simulink model "gm_PWMdutyFreqDetection"  (R2020b)
settings: Solver=FixedStepDiscrete  StartTime=0.0  StopTime=300e-6  RelTol=1e-3
libraries: simulink x4, hdlsllib x1
settings Model: Creator=Michael Hoerner  LastModifiedBy=Michael Hoerner
settings DataIOCC: LimitDataPoints=on  SaveOutput=off  SaveTime=off  ReturnWorkspaceOutputs=off
settings OptimizationCC: BlockReduction=off  ConditionallyExecuteInputs=off  DefaultParameterBehavior=Inlined  LifeSpan=inf
settings DebuggingCC: AlgebraicLoopMsg=error  InheritedTsInSrcMsg=none  SingleTaskRateTransMsg=warning  AllowSymbolicDim=off  StrictBusMsg=ErrorOnBusTreatedAsVector  SFUnexpectedBacktrackingDiag=warning  SFNoUnconditionalDefaultTransitionDiag=warning  SFExecutionAtInitializationDiag=none  ArithmeticOperatorsInVariantConditions=warning
settings HardwareCC: ProdBitPerPointer=32  ProdBitPerSizeT=32  ProdBitPerPtrDiffT=32  ProdLargestAtomicFloat=None  ProdIntDivRoundTo=Undefined  ProdEndianess=Unspecified  ProdWordSize=32  ProdHWDeviceType=ASIC/FPGA->ASIC/FPGA  ProdEqTarget=off
settings SFSimCC: SimUseLocalCustomCode=off  CustomCodeUndefinedFunction=UseInterfaceOnly
settings RTWCC: RTWUseLocalCustomCode=off
settings CodeAppCC: StateflowObjectComments=on
settings GRTTargetCC: TargetLangStandard=C89/C90 (ANSI)
settings ConfigComp: CovScope=ReferencedModels  CovMetricSettings=dw  CovSaveCumulativeToWorkspaceVar=on  CovSaveSingleToWorkspaceVar=on  CovExternalEMLEnable=off  CovSFcnEnable=off

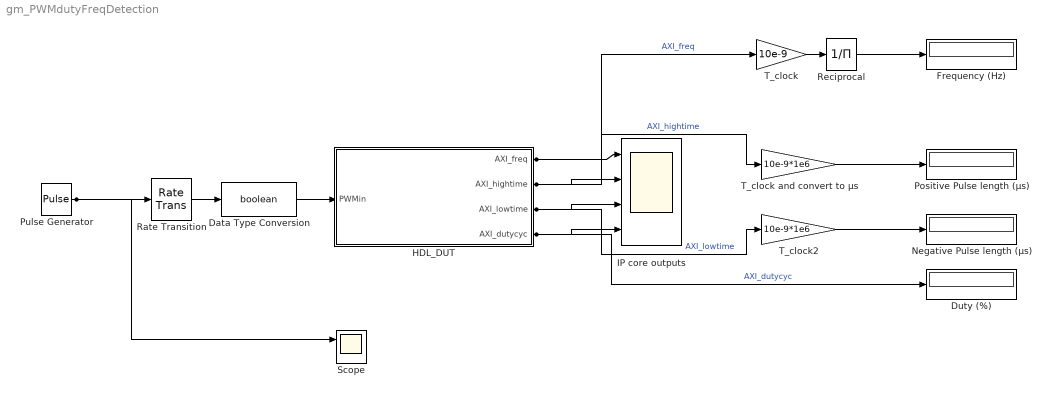
== system gm_PWMdutyFreqDetection ==
  Data Type Conversion : DataTypeConversion  OutDataTypeStr=boolean
  Duty (%) : Display
  Frequency (Hz) : Display
  HDL_DUT : Subsystem  TreatAsAtomicUnit=on
  IP core outputs : Scope  NumInputPorts=4
  Negative Pulse length (µs) : Display
  Positive Pulse length (µs) : Display
  Pulse Generator : DiscretePulseGenerator  PulseType=Time based  Period=1/10000  PulseWidth=25
  Rate Transition : RateTransition  OutPortSampleTime=10e-9
  Reciprocal : Product  Inputs=/
  Scope : Scope  NumInputPorts=2
  T_clock : Gain  Gain=10e-9
  T_clock and convert to µs : Gain  Gain=10e-9*1e6
  T_clock2 : Gain  Gain=10e-9*1e6
  wires:
  T_clock2/1 -> Negative Pulse length (µs)/1
  T_clock and convert to µs/1 -> Positive Pulse length (µs)/1
  Reciprocal/1 -> Frequency (Hz)/1
  T_clock/1 -> Reciprocal/1
  Data Type Conversion/1 -> HDL_DUT/1(PWMin)
  HDL_DUT/4(AXI_dutycyc) -> Duty (%)/1, IP core outputs/4  "AXI_dutycyc"
  HDL_DUT/3(AXI_lowtime) -> T_clock2/1, IP core outputs/3  "AXI_lowtime"
  HDL_DUT/2(AXI_hightime) -> IP core outputs/2, T_clock and convert to µs/1  "AXI_hightime"
  HDL_DUT/1(AXI_freq) -> IP core outputs/1, T_clock/1  "AXI_freq"
  Pulse Generator/1 -> Rate Transition/1, Scope/1
  Rate Transition/1 -> Data Type Conversion/1

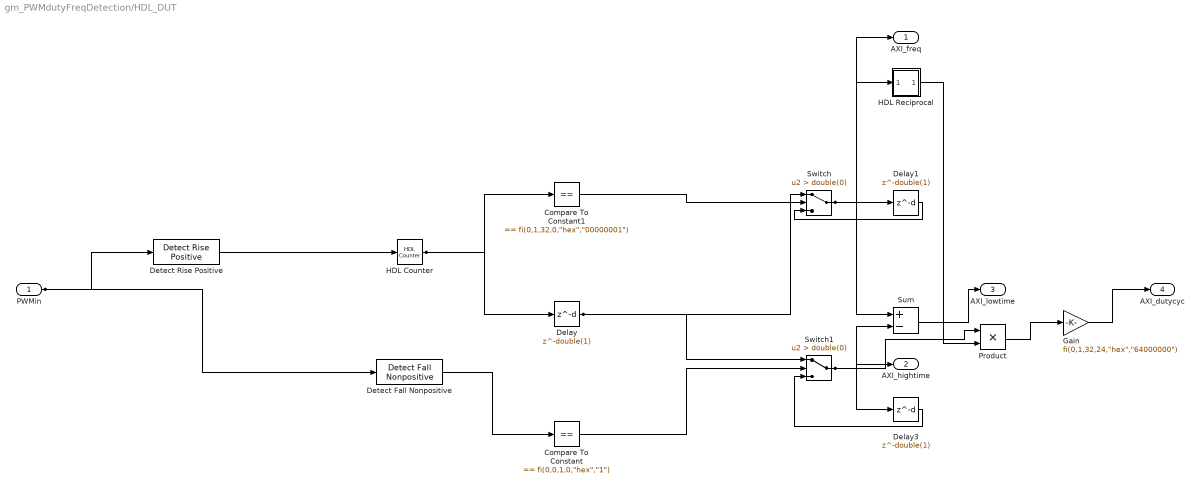
== system gm_PWMdutyFreqDetection/HDL_DUT ==
  PWMin : Inport  OutDataTypeStr=boolean  PortDimensions=1  SampleTime=1e-08
  Compare To Constant : simulink/Logic and Bit Operations/Compare To Constant  relop===  const="fi(0,0,1,0,\"hex\",\"1\")"  OutDataTypeStr=boolean
  Compare To Constant1 : simulink/Logic and Bit Operations/Compare To Constant  relop===  const="fi(0,1,32,0,\"hex\",\"00000001\")"  OutDataTypeStr=boolean
  Delay : Delay  DelayLength=double(1)  InitialCondition=0  SampleTime=1e-08
  Delay1 : Delay  DelayLength=double(1)  InitialCondition=0  SampleTime=1e-08
  Delay3 : Delay  DelayLength=double(1)  InitialCondition=0  SampleTime=1e-08
  Detect Fall Nonpositive : simulink/Logic and Bit Operations/Detect Fall Nonpositive  vinit=0  OutDataTypeStr=boolean
      settings: SourceProductBaseCode=SL
  Detect Rise Positive : simulink/Logic and Bit Operations/Detect Rise Positive  vinit=0  OutDataTypeStr=boolean
  Gain : Gain  Gain="fi(0,1,32,24,\"hex\",\"64000000\")"  ParamDataTypeStr=fixdt(1, 32, 24)  OutDataTypeStr=fixdt(1, 32, 24)  SampleTime=1e-08
  HDL Counter : hdlsllib/Sources/HDL Counter  CountType=Count limited  CountInit=double(1)  CountStep=double(1)  CountMax=double(2500000)  CountFromType=Initial value  CountFrom=double(1)  CountResetPort=on  CountLoadPort=off  CountEnbPort=off  CountDirPort=off  CountDataType=Signed  CountWordLen=32  CountFracLen=0  CountSampTime=1e-08
  HDL Reciprocal : Subsystem
  Product : Product  Inputs=**  OutDataTypeStr=fixdt(1, 32, 30)  SampleTime=1e-08
  Sum : Sum  Inputs=+-  AccumDataTypeStr=int32  OutDataTypeStr=int32  SampleTime=1e-08
  Switch : Switch  Criteria=u2 > Threshold  Threshold=double(0)  OutDataTypeStr=int32  SampleTime=1e-08
  Switch1 : Switch  Criteria=u2 > Threshold  Threshold=double(0)  OutDataTypeStr=int32  SampleTime=1e-08
  AXI_freq : Outport  VectorParamsAs1DForOutWhenUnconnected=off
  AXI_hightime : Outport  Port=2  VectorParamsAs1DForOutWhenUnconnected=off
  AXI_lowtime : Outport  Port=3  VectorParamsAs1DForOutWhenUnconnected=off
  AXI_dutycyc : Outport  Port=4  VectorParamsAs1DForOutWhenUnconnected=off
  wires:
  PWMin/1 -> Detect Fall Nonpositive/1, Detect Rise Positive/1
  Compare To Constant/1 -> Switch1/2
  Compare To Constant1/1 -> Switch/2
  Delay/1 -> Switch/1, Switch1/1
  Detect Fall Nonpositive/1 -> Compare To Constant/1
  Detect Rise Positive/1 -> HDL Counter/1
  Gain/1 -> AXI_dutycyc/1
  HDL Counter/1 -> Compare To Constant1/1, Delay/1
  HDL Reciprocal/1(Out1) -> Product/2
  Product/1 -> Gain/1
  Sum/1 -> AXI_lowtime/1
  Switch/1 -> Sum/1, HDL Reciprocal/1(In1), AXI_freq/1, Delay1/1
  Switch1/1 -> Sum/2, Product/1, AXI_hightime/1, Delay3/1
  Delay1/1 -> Switch/3
  Delay3/1 -> Switch1/3

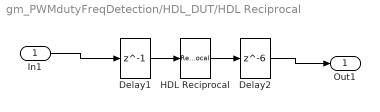
== system gm_PWMdutyFreqDetection/HDL_DUT/HDL Reciprocal ==
  In1 : Inport
  Delay1 : Delay  DelayLength=1
  Delay2 : Delay  DelayLength=6
  HDL Reciprocal : Reciprocal  SampleTime=1e-08
  Out1 : Outport
  wires:
  In1/1 -> Delay1/1
  Delay1/1 -> HDL Reciprocal/1
  HDL Reciprocal/1 -> Delay2/1
  Delay2/1 -> Out1/1
